simulink library "vmc"  (R2021b)
settings: Solver=VariableStepAuto  StartTime=0.0  StopTime=10.0  RelTol=1e-3
undefined symbols (not defined in the file or in its folder): AVMC_ACCDeltaTqIGain_X_kph, AVMC_ACCDeltaTqIGain_Y_mps2, AVMC_ACCDeltaTqIGainP2_X_kph, AVMC_ACCDeltaTqIGainP2_Y_mps2, AVMC_ACCDeltaTqPGain_X_kph, AVMC_ACCDeltaTqPGain_Y_kph, AVMC_ACCDeltaTqPGainP2_X_kph, AVMC_ACCDeltaTqPGainP2_Y_kph, AVMC_ACCLongSteadyCtrl_X_kph, AVMC_CCAccelCMD_X_kph, AVMC_CCAccelCMD_Y_kph, AVMC_CCDeltaTqIGain_X_kph, AVMC_CCDeltaTqIGain_Y_mps2, AVMC_CCDeltaTqPGain_X_kph, AVMC_CCDeltaTqPGain_Y_kph, AVMC_CCLongSteadyCtrl_X_kph, AVMC_DISCDeltaTqIGainP2_X_kph, AVMC_DISCDeltaTqIGainP2_Y_mps2, AVMC_ESCRegenOut_X_kph, AVMC_ESCRegenOut_Y_Deg, AVMC_ESCRegenOutEnSpd_X_Deg, AVMC_LatESCRegenOut_X_kph, AVMC_LatESCRegenOut_Y_Deg, AVMC_LongAccDeadZone_X_kph, AVMC_LongAccDeadZoneP2_X_kph, AVMC_LongAccFiltTs_X_Gps, AVMC_LongAccFiltTsP2_X_Gps, AVMC_MCPresBaseTq_X_bar, AVMC_MSAAccelCMD_X_kph, AVMC_MSAAccelCMD_Y_kph, AVMC_MSADeltaTqIGain_X_kph, AVMC_MSADeltaTqIGain_Y_mps2, AVMC_MSADeltaTqPGain_X_kph, AVMC_MSADeltaTqPGain_Y_kph, AVMC_MSALongSteadyCtrl_X_kph, AVMC_MSAPedalOvrd_X_kph, AVMC_MSASpdBand_X_kph, AVMC_OPDDisSlideRate_X_Deg, AVMC_RDCDetectTime_X_kph, AVMC_RDCDetectTime_Y_pct, AVMC_RDCEnSlideRate_X_Deg, AVMC_StESCYaw_X_kph, AVMC_StESCYaw_Y_Deg, AVMC_StESCYawCom_X_kph, AVMC_StESCYawCom_Y_Gps, AVMC_TMSpdBaseTq_X_rpm, C_TASK_10MS_S, C_TASK_5MS_S, DEG2RAD, Discrete, ENUM_ADASACCSTA_ACTIVE, ENUM_ADASACCSTA_OVERRIDE, ENUM_ADASACCSTA_STANDBY, ENUM_ADASMSASTA_ACTIVE, ENUM_ADASMSASTA_ERROR, ENUM_ADASMSASTA_OFF, ENUM_ADASMSASTA_OVERSPEED, ENUM_ADASMSASTA_STANDBY, ENUM_ADASMSASTA_UNDERSPEED, ENUM_ADASMSASTA_UNLIMIT ... (+254)
libraries: hcu_lib x57, simulink x49, ctrlSharedLib x6, simulink_extras x1
(part 7 of 9)

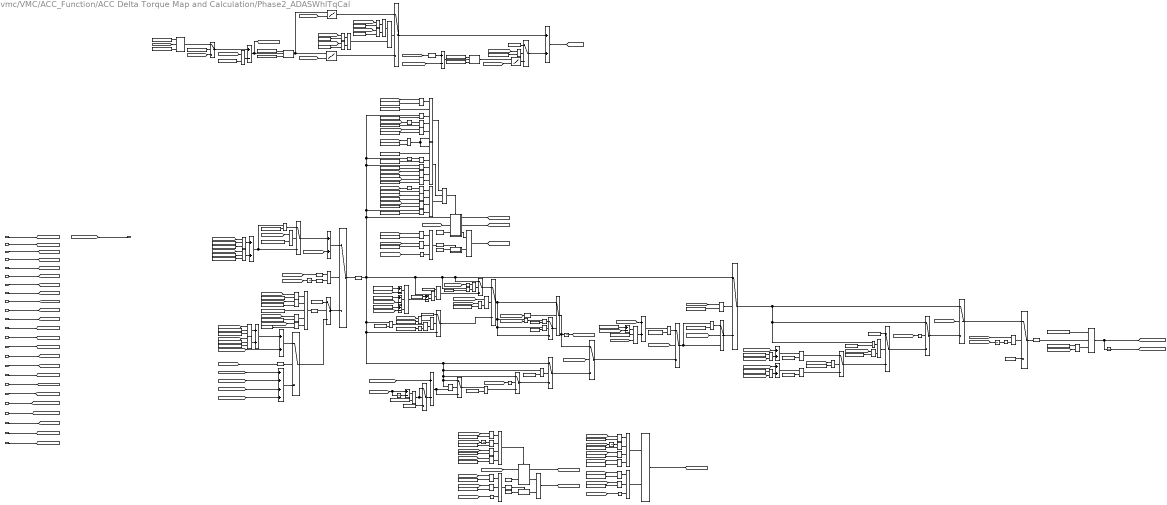
== system vmc/VMC/ACC_Function/ACC Delta Torque Map and Calculation/Phase2_ADASWhlTqCal ==
  note: Deceleration REGEN Torque Control
  note: Deceleration REGEN Torque Control Judgement
  note: Deceleration Torque Control
  note: Deceleration Positive Torque Control
  VVMC_TotalAvailBrkRgnTq_Nm : Inport
  VVMC_AccelTurnHold_flg : Inport  Port=2
  VVMC_ADASActive_flg : Inport  Port=3
  VVMC_ACCPedalOvrd_flg : Inport  Port=4
  task_time_s : Inport  Port=5
  VINP_ESCADASSta_enum : Inport  Port=6
  VVMC_MCPreBaseTqEn_flg : Inport  Port=7
  VINP_ACCVehHoldReq_flg : Inport  Port=8
  VINP_VehSpeed_kph : Inport  Port=9
  VINP_MCPressure_bar : Inport  Port=10
  VVMC_ADASNegReq_flg : Inport  Port=11
  VVMC_TimeGapJudge_flag : Inport  Port=12
  VTQR_FrTMTqReq_Nm : Inport  Port=13
  VTQR_RrTMTqReq_Nm : Inport  Port=14
  VVMC_LongAcc_Gps : Inport  Port=15
  VVMC_FeatSetSpdForCalcu_kph : Inport  Port=16
  VVMC_MeterIndSpeedForCalcu_kph : Inport  Port=17
  VINP_ADASACCSta_enum : Inport  Port=18
  VVMC_AfterCtrlACCReqAccel_mps2 : Inport  Port=19
  VVMC_TMSpdBaseTq_Nm : Inport  Port=20
  VVMC_MCPresBaseTq_Nm : Inport  Port=21
  VVMC_EstSlope_Deg : Inport  Port=22
  VVMC_ACCReqSpdMemory_kph : Inport  Port=23
  VVMC_ACCSpdCtrl_flg : Inport  Port=24
  AND{10,13,17,20,29,31} (6 alike) : Logic  AllPortsSameDT=off  OutDataTypeStr=boolean
  AND14 : Logic  Operator=OR  AllPortsSameDT=off  OutDataTypeStr=boolean
  AND19 : Logic  Operator=OR  AllPortsSameDT=off  OutDataTypeStr=boolean
  AND32 : Logic  Inputs=5  AllPortsSameDT=off  OutDataTypeStr=boolean
  Add{1,3,13,15,18..21} (8 alike) : Sum
  Add{4..5,7..12,14} (9 alike) : Sum  Inputs=+-
  Add6 : Sum  Inputs=++++
  Cast To Single2 : DataTypeConversion  OutDataTypeStr=single
  Cast To Single3 : DataTypeConversion  OutDataTypeStr=single
  Constant1 : Constant  Value=ENUM_ADASACCSTA_ACTIVE
  Constant10 : Constant  Value=KVMC_ADASWhlTqLowerLim_Nm
  Constant100 : Constant  Value=KVMC_ZeroRgnTqSpdCtrlTime_s
  Constant{30,42..43,46,48,53..56,58,63..64,66..67,69..70,72..75,81..82,87,89..90,92..93,96,98..99,101,112,114,116..117,124..125,131..132,151,156,163,168,170,174} (45 alike) : Constant  Value=ZERO_FLOAT
  Constant11 : Constant  Value=KVMC_ReqAccelLimitSW_flg
  Constant115 : Constant  Value=KVMC_ACCLowSpdPosTq_flg
  Constant12 : Constant  Value=KVMC_AccDevLowLim_mps2
  Constant13 : Constant  Value=KVMC_AccDevUpLim_mps2
  Constant14 : Constant  Value=KVMC_ACCSpdDevUpLim_kph
  Constant15 : Constant  Value=KVMC_ACCSpdDevLowLim_kph
  Constant157 : Constant  Value=KVMC_AccelTurnHoldZeroTq_flg
  Constant16 : Constant  Value=KVMC_ReqAccelUpperLimit_mps2
  Constant162 : Constant  Value=KVMC_HoldTqRamp2ZeroSlope_Nmps
  Constant166 : Constant  Value=ENUM_ESCADASSTA_VEHASTANDSTILL
  Constant167 : Constant  Value=KVMC_StandstillTqRamp2ZeroSlope_Nmps
  Constant17 : Constant  Value=KVMC_ReqAccelLowerLimit_mps2
  Constant171 : Constant  Value=KVMC_BigDeltaDecGapBand_mps2
  Constant172 : Constant  Value=KVMC_BigDeltaDecJudgeEnBand_mps2
  Constant173 : Constant  Value=KVMC_BigDeltaDecEnGradeBand_deg
  Constant2 : Constant  Value=KTQR_FrTMGearEff_c
  Constant23 : Constant  Value=TRUE
  Constant27 : Constant  Value=KVMC_TimeGapTq2Zero_flg
  Constant3 : Constant  Value=KTQD_FrTMTotalGearRatio_gain
  Constant{38..39,57,62,77,80,88,97} (8 alike) : Constant  Value=KVMC_CutOffNegTqSpd_kph
  Constant4 : Constant  Value=KTQD_RrTMTotalGearRatio_gain
  Constant40 : Constant  Value=KTQR_FrTMGearEff_c
  Constant41 : Constant  Value=FALSE
  Constant{44,50..51,78..79,91} (6 alike) : Constant  Value=KVMC_ZeroRgnTqSpd_kph
  Constant45 : Constant  Value=KTQD_FrTMTotalGearRatio_gain
  Constant5 : Constant  Value=KTQR_RrTMGearEff_c
  Constant59 : Constant  Value=KVMC_TqMCPRelFactor_Nm
  Constant68 : Constant  Value=KVMC_GradeTqCtrl_flg
  Constant71 : Constant  Value=KVMC_BigDeltaDecGapZeroTq_flg
  Constant76 : Constant  Value=KVMC_DownGradeTqCtrl_flg
  Constant8 : Constant  Value=KVMC_ADASWhlTqUpperLim_Nm
  Constant84 : Constant  Value=KTQD_RrTMTotalGearRatio_gain
  Constant85 : Constant  Value=KTQR_RrTMGearEff_c
  Constant9 : Constant  Value=KVMC_GravityValue_mps2
  Constant94 : Constant  Value=TRUE
  Constant95 : Constant  Value=FALSE
  Data Type Conversion1 : DataTypeConversion  OutDataTypeStr=single
  Detect Decrease2 : simulink/Logic and Bit Operations/Detect Decrease  vinit=0.0  OutDataTypeStr=boolean
  Detect Decrease3 : simulink/Logic and Bit Operations/Detect Decrease  vinit=0.0  OutDataTypeStr=boolean
  Detect Increase{3..5,7..8} (5 alike) : simulink/Logic and Bit Operations/Detect Increase  vinit=0.0  OutDataTypeStr=boolean
  Divide : Product  Inputs=*/*
  Divide{1,4..5,8} (4 alike) : Product  Inputs=***
  Divide2 : Product  Inputs=**
  Divide3 : Product  Inputs=*/*
  Divide6 : Product  Inputs=**
  Divide7 : Product  Inputs=**
  Equal10 : RelationalOperator  Operator===  OutDataTypeStr=boolean  RndMeth=Simplest
  Equal11 : RelationalOperator  Operator=<  OutDataTypeStr=boolean  RndMeth=Simplest
  Equal12 : RelationalOperator  Operator=>  OutDataTypeStr=boolean  RndMeth=Simplest
  Equal6 : RelationalOperator  Operator=<  OutDataTypeStr=boolean  RndMeth=Simplest
  Equal7 : RelationalOperator  Operator=>  OutDataTypeStr=boolean  RndMeth=Simplest
  Equal8 : RelationalOperator  Operator=<  OutDataTypeStr=boolean  RndMeth=Simplest
  Equal9 : RelationalOperator  Operator=>  OutDataTypeStr=boolean  RndMeth=Simplest
  InitialCondition: 1 : UnitDelay  SampleTime=-1  HasFrameUpgradeWarning=on
  Logical Operator1 : Logic  Inputs=4  AllPortsSameDT=off  OutDataTypeStr=boolean
  Logical Operator10 : Logic  Operator=OR  Inputs=3  AllPortsSameDT=off  OutDataTypeStr=boolean
  Logical Operator2 : Logic  Operator=OR  AllPortsSameDT=off  OutDataTypeStr=boolean
  Logical Operator3 : Logic  Inputs=6  AllPortsSameDT=off  OutDataTypeStr=boolean
  Logical Operator4 : Logic  Operator=OR  Inputs=3  AllPortsSameDT=off  OutDataTypeStr=boolean
  Logical Operator5 : Logic  Inputs=6  AllPortsSameDT=off  OutDataTypeStr=boolean
  Logical Operator6 : Logic  AllPortsSameDT=off  OutDataTypeStr=boolean
  Logical Operator7 : Logic  Inputs=4  AllPortsSameDT=off  OutDataTypeStr=boolean
  Logical Operator8 : Logic  Operator=OR  Inputs=3  AllPortsSameDT=off  OutDataTypeStr=boolean
  Logical Operator9 : Logic  Inputs=4  AllPortsSameDT=off  OutDataTypeStr=boolean
  MVMC_ACCDeltaTqIGain_Z_Nm : Lookup_n-D  BreakpointsForDimension1=AVMC_ACCDeltaTqIGainP2_Y_mps2  BreakpointsForDimension2=AVMC_ACCDeltaTqIGainP2_X_kph  Table=MVMC_ACCDeltaTqIGainP2_Z_Nm  InternalRulePriority=Speed  RndMeth=Simplest  InputSameDT=on
      settings: InputPortMap=u0,u1
  MVMC_ACCDeltaTqPGain_Z_Nm1 : Lookup_n-D  BreakpointsForDimension1=AVMC_ACCDeltaTqPGainP2_Y_kph  BreakpointsForDimension2=AVMC_ACCDeltaTqPGainP2_X_kph  Table=MVMC_ACCDeltaTqPGainP2_Z_Nm  InternalRulePriority=Speed  RndMeth=Simplest  InputSameDT=on
      settings: InputPortMap=u0,u1
  MVMC_DISCDeltaTqIGain_Z_Nm : Lookup_n-D  BreakpointsForDimension1=AVMC_DISCDeltaTqIGainP2_Y_mps2  BreakpointsForDimension2=AVMC_DISCDeltaTqIGainP2_X_kph  Table=MVMC_DISCDeltaTqIGainP2_Z_Nm  InternalRulePriority=Speed  RndMeth=Simplest  InputSameDT=on
      settings: InputPortMap=u0,u1
  Max{,1,4..5,7..8} (6 alike) : MinMax  Function=max  Inputs=2
  Max2 : MinMax  Inputs=2
  Max3 : MinMax  Inputs=2
  Merge : Merge
  Merge2 : Merge
  Min : MinMax  Inputs=2
  Min1 : MinMax  Inputs=2
  Min2 : MinMax  Function=max  Inputs=2
  NOT{1,4..6,9,12..13,15} (8 alike) : Logic  Operator=NOT  AllPortsSameDT=off  OutDataTypeStr=boolean
  OR18 : Logic  Operator=OR  AllPortsSameDT=off  OutDataTypeStr=boolean
  OR2 : Logic  Operator=OR  Inputs=3  AllPortsSameDT=off  OutDataTypeStr=boolean
  OR5 : Logic  AllPortsSameDT=off  OutDataTypeStr=boolean
  Product1 : Product
  Relational Operator1 : RelationalOperator  Operator=~=  OutDataTypeStr=boolean  RndMeth=Simplest
  Relational Operator{2,10,12,24..25,29,36..37,39,42..43} (11 alike) : RelationalOperator  OutDataTypeStr=boolean  RndMeth=Simplest
  Relational Operator{9,11,14..15,21..23,26,28,30..31,35,41,45,49..50} (16 alike) : RelationalOperator  Operator=<  OutDataTypeStr=boolean  RndMeth=Simplest
  Relational Operator{20,27,34,40,71,74} (6 alike) : RelationalOperator  Operator=<=  OutDataTypeStr=boolean  RndMeth=Simplest
  Relational Operator{32..33,38,44,47} (5 alike) : RelationalOperator  Operator=>  OutDataTypeStr=boolean  RndMeth=Simplest
  SR_Latch : hcu_lib/Basic_Blocks/SR_Latch
  Saturation Dynamic{1..3,5} (4 alike) : simulink/Discontinuities/Saturation Dynamic  OutMin=[]  OutMax=[]  OutDataTypeStr=Inherit: Same as second input  OutDataType=fixdt(1, 16)  OutScaling=2^-10  DoSatur=off
  Switch{,1,4,7..8,10,12..19,21..24,27,29,33..34,39,41,43} (25 alike) : Switch  Criteria=u2 > Threshold
  Triggered Subsystem1 : Subsystem  TreatAsAtomicUnit=on
  Triggered Subsystem2 : Subsystem  TreatAsAtomicUnit=on
  Triggered Subsystem4 : Subsystem  TreatAsAtomicUnit=on
  Triggered Subsystem5 : Subsystem  TreatAsAtomicUnit=on
  Unit Delay{1..5,7..9,11} (9 alike) : UnitDelay  SampleTime=-1  HasFrameUpgradeWarning=on
  VVMC_ADASWhlTqCal_Nm : Outport
  wires:
  Constant66/1 -> Relational Operator23/2
  Relational Operator42/1 -> Logical Operator9/2
  Detect Increase3/1 -> Triggered Subsystem2/Trigger
  Detect Decrease3/1 -> Logical Operator2/2
  Unit Delay2/1 -> Detect Decrease3/1
  NOT13/1 -> AND10/1
  Max2/1 -> Switch24/1
  Relational Operator30/1 -> Logical Operator5/3
  Relational Operator44/1 -> Logical Operator10/1
  [VTQR_RrTMTqReq_Nm] -> Divide5/1
  Constant162/1 -> Divide6/1
  NOT6/1 -> OR5/2
  Switch19/1 -> Switch18/3
  Relational Operator47/1 -> AND10/2
  Constant112/1 -> Relational Operator47/2
  Max4/1 -> Min1/2
  Constant99/1 -> Add14/1
  Constant68/1 -> Logical Operator3/2
  [VVMC_ACCLowSpdCtrlEnSpd_kph] -> Relational Operator33/1
  NOT15/1 -> Logical Operator10/3
  Constant39/1 -> Relational Operator12/2
  Constant77/1 -> Relational Operator31/2
  Merge2/1 -> [VVMC_ZeroRgnTqSpdCtrl_flg]  "VVMC_ZeroRgnTqSpdCtrl_flg"
  Relational Operator38/1 -> Logical Operator8/1
  Switch17/1 -> Relational Operator71/1, Switch13/1, Switch4/1
  Constant115/1 -> NOT12/1
  Constant46/1 -> Min/2
  [VVMC_ActACCRequiredAccel_mps2] -> Unit Delay7/1
  Cast To Single2/1 -> Relational Operator9/1, Switch10/1, Switch16/1, Relational Operator26/1, Switch19/1, Switch21/3, Relational Operator49/1, Relational Operator30/1, Unit Delay4/1, Relational Operator23/1, Relational Operator15/1, Triggered Subsystem1/1(In1), Max4/1, Relational Operator47/1, Switch27/1, Switch17/1  "VVMC_OriADASWhlTqP2_Nm"
  Relational Operator39/1 -> Logical Operator7/1
  Unit Delay8/1 -> [VVMC_LastACCLowSpdTq_Nm]
  Divide6/1 -> Add20/2
  [VVMC_ZeroRgnTqSpdCtrlTq_Nm] -> Add14/2
  Constant93/1 -> Relational Operator42/2
  Relational Operator22/1 -> Logical Operator3/6
  Constant44/1 -> Relational Operator20/2
  Relational Operator27/1 -> AND32/1
  Add9/1 -> Divide/2
  Constant90/1 -> Relational Operator39/2
  Equal10/1 -> Switch41/2
  Add21/1 -> Max8/1
  [VVMC_ADASActive_flg] -> NOT4/1
  Add14/1 -> Divide3/1
  Switch41/1 -> Switch39/3
  Relational Operator43/1 -> Logical Operator10/2
  Detect Increase5/1 -> Switch22/2
  [VVMC_LastADASWhlTqCal_Nm] -> Relational Operator39/1
  InitialCondition: 1/1 -> [VVMC_LastADASWhlTqCal_Nm]  "VVMC_LastADASWhlTqCalP2_Nm"
  Relational Operator12/1 -> Logical Operator1/1
  OR2/1 -> Triggered Subsystem1/Trigger
  Divide3/1 -> Add15/2
  Constant151/1 -> Relational Operator71/2
  Triggered Subsystem1/3(Out3) -> Merge/1
  [VINP_VehSpeed_kph] -> Relational Operator38/1
  Add8/1 -> Divide/1
  AND29/1 -> OR18/2
  Constant95/1 -> Triggered Subsystem5/1(In1)
  Constant97/1 -> Relational Operator44/2
  Max3/1 -> Switch29/1
  Detect Increase8/1 -> Switch43/2
  [VVMC_ActACCRequiredAccel_mps2] -> Relational Operator43/1
  Triggered Subsystem2/1(Out1) -> Merge/2
  Constant89/1 -> Max1/2
  [VVMC_ADASActive_flg] -> NOT15/1
  Switch39/1 -> Switch13/3
  Triggered Subsystem5/1(Out1) -> Merge2/2
  Constant53/1 -> Add10/1
  Switch23/1 -> Switch17/3
  Relational Operator28/1 -> Logical Operator5/5
  Constant57/1 -> Relational Operator2/2
  Constant98/1 -> Relational Operator45/2
  [VVMC_ActACCRequiredAccel_mps2] -> Relational Operator14/1
  Add18/1 -> Switch8/1
  Constant48/1 -> Relational Operator15/2
  Switch43/1 -> Switch8/3
  [task_time_s] -> Divide7/2
  AND31/1 -> Switch33/2
  Switch33/1 -> Add18/1
  [VVMC_ADASActive_flg] -> Detect Increase4/1
  [VTQR_FrTMTqReq_Nm] -> Divide1/1
  Switch4/1 -> Switch7/1
  Relational Operator32/1 -> Logical Operator5/6, Logical Operator3/1
  [VINP_VehSpeed_kph] -> Relational Operator44/1
  AND10/1 -> Switch27/2
  [VVMC_ActACCRequiredAccel_mps2] -> Relational Operator28/1
  [VVMC_ADASNegReq_flg] -> NOT13/1
  [VINP_VehSpeed_kph] -> Relational Operator2/1
  [VVMC_ActACCRequiredAccel_mps2] -> Relational Operator22/1
  Relational Operator29/1 -> Logical Operator5/4
  Add20/1 -> Max7/1
  NOT9/1 -> Logical Operator8/3
  [VVMC_ACCPedalOvrd_flg] -> Unit Delay2/1
  Relational Operator45/1 -> Logical Operator9/1
  [VINP_VehSpeed_kph] -> Unit Delay1/1
  [VVMC_AccelTurnHold_flg] -> AND29/1
  AND14/1 -> AND13/2
  Max8/1 -> Switch41/1
  [VINP_ESCADASSta_enum] -> Equal10/1
  Constant96/1 -> Relational Operator43/2
  [VINP_VehSpeed_kph] -> Relational Operator32/1
  Constant114/1 -> Relational Operator49/2
  [VVMC_EstSlope_Deg] -> Equal11/1
  Max/1 -> Max3/1
  Constant116/1 -> Relational Operator50/2
  Constant73/1 -> Relational Operator29/2
  Relational Operator15/1 -> Logical Operator1/4
  Switch21/1 -> Switch12/3
  Constant172/1 -> Relational Operator74/2
  Constant84/1 -> Divide5/2
  Constant92/1 -> Relational Operator41/2
  Unit Delay1/1 -> Relational Operator12/1
  Divide5/1 -> Add13/2
  Logical Operator10/1 -> Detect Increase7/1
  [VVMC_ACCLowSpdTqCtrl_flg] -> Detect Increase5/1
  Triggered Subsystem1/1(Out1) -> [VVMC_ACCLowSpdTqLimit_Nm]  "VVMC_ACCLowSpdTqLimit_Nm"
  Saturation Dynamic2/1 -> [VVMC_ADASWhlTqCal_Nm], InitialCondition: 1/1  "VVMC_ADASWhlTqCalP2_Nm"
  OR5/1 -> Switch7/2
  Relational Operator33/1 -> Logical Operator6/2
  Divide/1 -> Add4/2
  Relational Operator50/1 -> Switch29/2
  Min1/1 -> Switch27/3
  [VVMC_ActACCRequiredAccel_mps2] -> Relational Operator37/1
  Add6/1 -> Switch14/3
  Logical Operator2/1 -> Switch8/2
  Switch29/1 -> Switch22/3
  OR18/1 -> Switch39/2
  Logical Operator6/1 -> Switch12/2
  Constant170/1 -> Switch43/1
  Switch8/1 -> Cast To Single2/1
  Constant80/1 -> Relational Operator34/2
  Constant42/1 -> Relational Operator24/2
  Unit Delay9/1 -> Relational Operator36/1
  [VINP_VehSpeed_kph] -> Relational Operator20/1
  Relational Operator74/1 -> AND32/2
  Relational Operator41/1 -> Logical Operator9/3
  Switch12/1 -> Switch29/3, Relational Operator50/1, Max/1, Switch22/1
  Relational Operator36/1 -> Logical Operator7/2
  [VINP_VehSpeed_kph] -> Relational Operator11/1
  [VVMC_TimeGapJudge_flag] -> AND31/1
  NOT4/1 -> Logical Operator4/3
  [task_time_s] -> Divide3/3
  Relational Operator71/1 -> OR18/1
  Constant75/1 -> Relational Operator30/2
  [VINP_VehSpeed_kph] -> Relational Operator31/1
  [VINP_VehSpeed_kph] -> Relational Operator34/1
  Relational Operator49/1 -> AND14/1
  Constant76/1 -> Logical Operator5/2
  Constant166/1 -> Equal10/2
  Detect Increase4/1 -> Logical Operator2/1
  Constant74/1 -> Switch7/3
  Constant64/1 -> Relational Operator22/2
  Constant40/1 -> Divide1/3
  Divide7/1 -> Add21/2
  [VINP_VehSpeed_kph] -> Relational Operator21/1
  Logical Operator3/1 -> OR2/2
  Constant163/1 -> Max7/2
  Constant54/1 -> Add4/1
  [task_time_s] -> Divide6/2
  Constant82/1 -> Relational Operator36/2
  [VINP_ACCVehHoldReq_flg] -> NOT5/1
  [VVMC_LastADASWhlTqCal_Nm] -> Add15/1
  Constant117/1 -> Max3/2
  [VVMC_ZeroRgnTqSpdCtrl_flg] -> Switch24/2
  Constant56/1 -> Switch21/1
  Constant23/1 -> Triggered Subsystem1/3(In3)
  [VINP_VehSpeed_kph] -> Relational Operator40/1
  Switch7/1 -> Cast To Single3/1
  Constant71/1 -> AND32/3
  Constant157/1 -> AND29/2
  [VVMC_ACCLowSpdCtrlEnSpd_kph] -> Add9/2
  NOT12/1 -> AND14/2
  Constant167/1 -> Divide7/1
  Constant55/1 -> Min1/1
  [VVMC_ActACCRequiredAccel_mps2] -> Relational Operator24/1
  Relational Operator31/1 -> Logical Operator5/1
  Logical Operator5/1 -> OR2/1
  Constant78/1 -> Relational Operator32/2
  Constant100/1 -> Divide3/2
  [VVMC_ACCDeltaTq_Nm] -> Add19/2
  [VVMC_MCPresBaseTq_Nm] -> Add6/4
  Constant101/1 -> Max2/2
  Constant174/1 -> Equal12/2
  Constant85/1 -> Divide5/3
  AND13/1 -> Switch21/2
  [VVMC_ACCDeltaTq_Nm] -> Add18/2
  [VVMC_TMSpdBaseTq_Nm] -> Add6/3
  Relational Operator37/1 -> Logical Operator8/2
  Relational Operator2/1 -> Logical Operator4/1
  Constant72/1 -> Relational Operator28/2
  Constant87/1 -> Relational Operator37/2
  AND32/1 -> Detect Increase8/1
  [VVMC_LastADASWhlTqCal_Nm] -> Add6/1
  Triggered Subsystem1/2(Out2) -> [VVMC_ACCLowSpdCtrlEnSpd_kph]  "VVMC_ACCLowSpdCtrlEnSpd_kph"
  Constant168/1 -> Max8/2
  Switch24/1 -> Switch23/3, Max1/1
  [VVMC_ACCPedalOvrd_flg] -> Unit Delay5/1
  Merge/1 -> [VVMC_ACCLowSpdTqCtrl_flg]  "VVMC_ACCLowSpdTqCtrl_flg"
  Relational Operator21/1 -> Logical Operator3/5
  Relational Operator24/1 -> Switch17/2
  Constant27/1 -> AND31/2
  Constant171/1 -> Relational Operator27/2
  Max7/1 -> Switch41/3
  [VVMC_ACCLowSpdTqCtrl_flg] -> Logical Operator6/1
  Constant156/1 -> Switch39/1
  Relational Operator35/1 -> Logical Operator7/3
  Switch27/1 -> Switch12/1
  [VVMC_ACCDeltaAccel_mps2] -> Relational Operator27/1
  Relational Operator11/1 -> Logical Operator1/2
  Relational Operator20/1 -> AND13/1
  [VVMC_LastADASWhlTqCal_Nm] -> Equal12/1
  [VVMC_LastADASWhlTqCal_Nm] -> Add21/1
  [VVMC_ADASActive_flg] -> NOT9/1
  [VVMC_LastACCLowSpdTq_Nm] -> Max/2
  [VVMC_RgnProhibited_flg] -> Switch23/2
  [VVMC_ActACCRequiredAccel_mps2] -> Unit Delay9/1
  [VVMC_LastADASWhlTqCal_Nm] -> Triggered Subsystem4/1(In1)
  Unit Delay7/1 -> Relational Operator29/1
  Switch22/1 -> Switch18/1, Unit Delay8/1  "VVMC_ACCLowSpdTq_Nm"
  Equal12/1 -> AND32/5
  Relational Operator25/1 -> Logical Operator3/3
  Constant81/1 -> Relational Operator35/2
  [VVMC_ActACCRequiredAccel_mps2] -> Relational Operator74/1
  Detect Decrease2/1 -> Switch14/2
  Triggered Subsystem4/2(Out2) -> Merge2/1
  [VVMC_ACCLowSpdTqCtrl_flg] -> Switch18/2
  Equal11/1 -> AND32/4
  [VVMC_ActACCRequiredAccel_mps2] -> Relational Operator35/1
  Constant43/1 -> Relational Operator14/2
  Switch13/1 -> Switch4/3
  Constant88/1 -> Relational Operator38/2
  [VVMC_ACCDeltaTq_Nm] -> Add6/2
  Relational Operator14/1 -> Logical Operator1/3
  [VVMC_MCPreBaseTqEn_flg] -> Switch4/2
  [VVMC_LastADASWhlTqCal_Nm] -> Add20/1
  Constant51/1 -> Add9/1
  [VVMC_ADASActive_flg] -> OR5/1
  Constant62/1 -> Relational Operator21/2
  [VVMC_ACCLowSpdTqLimit_Nm] -> Add10/2
  Add13/1 -> Min/1, Switch33/3
  SR_Latch/1 -> [VVMC_RgnProhibited_flg]  "VVMC_RgnProhibited_flg"
  Relational Operator40/1 -> Logical Operator9/4
  Triggered Subsystem4/1(Out1) -> [VVMC_ZeroRgnTqSpdCtrlTq_Nm]  "VVMC_ZeroRgnTqSpdCtrlTq_Nm"
  Relational Operator23/1 -> Logical Operator3/4
  Unit Delay4/1 -> Relational Operator25/1
  [VVMC_ActACCRequiredAccel_mps2] -> Relational Operator10/1
  [VINP_VehSpeed_kph] -> Triggered Subsystem1/2(In2)
  [VVMC_ActACCRequiredAccel_mps2] -> Unit Delay11/1
  Constant79/1 -> Relational Operator33/2
  Logical Operator4/1 -> Detect Increase3/1
  Logical Operator9/1 -> Triggered Subsystem4/Trigger
  Constant173/1 -> Equal11/2
  Constant41/1 -> Triggered Subsystem2/1(In1)
  Add4/1 -> Max4/2
  Divide1/1 -> Add13/1
  Constant91/1 -> Relational Operator40/2
  Add15/1 -> Max2/1
  Unit Delay11/1 -> Relational Operator42/1
  [VVMC_LastADASWhlTqCal_Nm] -> Relational Operator45/1
  Max1/1 -> Switch23/1
  Constant45/1 -> Divide1/2
  Switch14/1 -> Switch43/3
  Relational Operator34/1 -> Logical Operator7/4
  Add10/1 -> Divide/3
  Switch18/1 -> Switch24/3
  [VINP_VehSpeed_kph] -> Add8/2
  Constant94/1 -> Triggered Subsystem4/2(In2)
  NOT5/1 -> Switch13/2
  Constant67/1 -> Relational Operator25/2
  Add19/1 -> Switch14/1
  Constant50/1 -> Add8/1
  Detect Increase7/1 -> Triggered Subsystem5/Trigger
  Constant30/1 -> Relational Operator10/2
  Unit Delay5/1 -> NOT6/1
  Logical Operator1/1 -> OR2/3
  Relational Operator10/1 -> Logical Operator4/2
  Constant38/1 -> Relational Operator11/2
  [VVMC_ActACCRequiredAccel_mps2] -> Relational Operator41/1
  [VVMC_ADASNegReq_flg] -> Detect Decrease2/1
  VVMC_AccelTurnHold_flg/1 -> [VVMC_AccelTurnHold_flg]
  VVMC_TotalAvailBrkRgnTq_Nm/1 -> [VVMC_TotalAvailBrkRgnTq_Nm]
  [VVMC_ADASWhlTqCal_Nm] -> VVMC_ADASWhlTqCal_Nm/1
  VVMC_ADASActive_flg/1 -> [VVMC_ADASActive_flg]
  VVMC_ACCPedalOvrd_flg/1 -> [VVMC_ACCPedalOvrd_flg]
  task_time_s/1 -> [task_time_s]
  VINP_ESCADASSta_enum/1 -> [VINP_ESCADASSta_enum]
  VVMC_MCPreBaseTqEn_flg/1 -> [VVMC_MCPreBaseTqEn_flg]
  VINP_ACCVehHoldReq_flg/1 -> [VINP_ACCVehHoldReq_flg]
  VINP_VehSpeed_kph/1 -> [VINP_VehSpeed_kph]
  VINP_MCPressure_bar/1 -> [VINP_MCPressure_bar]
  VVMC_ADASNegReq_flg/1 -> [VVMC_ADASNegReq_flg]
  VVMC_TimeGapJudge_flag/1 -> [VVMC_TimeGapJudge_flag]
  VTQR_FrTMTqReq_Nm/1 -> [VTQR_FrTMTqReq_Nm]
  VTQR_RrTMTqReq_Nm/1 -> [VTQR_RrTMTqReq_Nm]
  Saturation Dynamic1/1 -> MVMC_DISCDeltaTqIGain_Z_Nm/1, MVMC_ACCDeltaTqIGain_Z_Nm/1  "VVMC_ActAccDevP2_mps2"
  Saturation Dynamic5/1 -> MVMC_ACCDeltaTqPGain_Z_Nm1/1  "VVMC_ACCActSpdDevP2_kph"
  MVMC_ACCDeltaTqPGain_Z_Nm1/1 -> Switch1/3
  AND20/1 -> AND19/2
  Constant9/1 -> Product1/2
  Constant12/1 -> Saturation Dynamic1/3
  Switch1/1 -> Add3/2  "VVMC_ACCDeltaTqPGainP2_Nm"
  Constant58/1 -> Switch1/1
  Relational Operator1/1 -> Switch1/2
  Add5/1 -> Saturation Dynamic5/2
  Data Type Conversion1/1 -> Add5/1
  [VVMC_ActACCRequiredAccel_mps2] -> Equal7/1
  [VVMC_LongAcc_Gps] -> Equal6/1
  [VVMC_MeterIndSpeedForCalcu_kph] -> Add5/2
  Constant15/1 -> Saturation Dynamic5/3
  [VVMC_FeatSetSpdForCalcu_kph] -> Data Type Conversion1/1
  AND19/1 -> Switch34/2
  [VINP_VehSpeed_kph] -> MVMC_ACCDeltaTqPGain_Z_Nm1/2
  Product1/1 -> Add7/2
  Constant131/1 -> Equal8/2
  Constant124/1 -> Equal6/2
  [VINP_VehSpeed_kph] -> MVMC_DISCDeltaTqIGain_Z_Nm/2
  Add7/1 -> [VVMC_ACCDeltaAccel_mps2], Saturation Dynamic1/2
  [VVMC_ACCDeltaAccel_mps2] -> Equal9/1
  Constant132/1 -> Equal9/2
  [VVMC_LongAcc_Gps] -> Product1/1
  Equal7/1 -> AND17/2
  Constant125/1 -> Equal7/2
  MVMC_DISCDeltaTqIGain_Z_Nm/1 -> Switch34/1
  MVMC_ACCDeltaTqIGain_Z_Nm/1 -> Switch34/3
  Constant14/1 -> Saturation Dynamic5/1
  [VVMC_ActACCRequiredAccel_mps2] -> Switch/3
  Switch34/1 -> Add3/1  "VVMC_ACCDeltaTqIGainP2_Nm"
  [VINP_VehSpeed_kph] -> MVMC_ACCDeltaTqIGain_Z_Nm/2
  Equal6/1 -> AND17/1
  Equal8/1 -> AND20/1
  Constant13/1 -> Saturation Dynamic1/1
  AND17/1 -> AND19/1
  Equal9/1 -> AND20/2
  Add3/1 -> [VVMC_ACCDeltaTq_Nm]  "VVMC_ACCDeltaTqP2_Nm"
  [VVMC_ActACCRequiredAccel_mps2] -> Equal8/1
  Constant1/1 -> Relational Operator1/2
  [VINP_ADASACCSta_enum] -> Relational Operator1/1
  VVMC_LongAcc_Gps/1 -> [VVMC_LongAcc_Gps]
  VVMC_FeatSetSpdForCalcu_kph/1 -> [VVMC_FeatSetSpdForCalcu_kph]
  VVMC_MeterIndSpeedForCalcu_kph/1 -> [VVMC_MeterIndSpeedForCalcu_kph]
  VINP_ADASACCSta_enum/1 -> [VINP_ADASACCSta_enum]
  VVMC_AfterCtrlACCReqAccel_mps2/1 -> [VVMC_ActACCRequiredAccel_mps2]
  VVMC_TMSpdBaseTq_Nm/1 -> [VVMC_TMSpdBaseTq_Nm]
  VVMC_MCPresBaseTq_Nm/1 -> [VVMC_MCPresBaseTq_Nm]
  Constant3/1 -> Divide4/2
  Divide4/1 -> Add1/1
  Constant5/1 -> Divide8/3
  Constant2/1 -> Divide4/3
  Divide8/1 -> Add1/2
  Constant4/1 -> Divide8/2
  [VTQR_FrTMTqReq_Nm] -> Divide4/1
  [VTQR_RrTMTqReq_Nm] -> Divide8/1
  Add1/1 -> Add19/1
  VVMC_EstSlope_Deg/1 -> [VVMC_EstSlope_Deg]
  VVMC_ACCReqSpdMemory_kph/1 -> [VVMC_ACCReqSpdMemory_kph]
  VVMC_ACCSpdCtrl_flg/1 -> [VVMC_ACCSpdCtrl_flg]
  [VVMC_TotalAvailBrkRgnTq_Nm] -> Max5/2
  Constant10/1 -> Max5/1
  Max5/1 -> Saturation Dynamic2/3
  Constant8/1 -> Saturation Dynamic2/1
  Cast To Single3/1 -> Saturation Dynamic2/2
  Constant11/1 -> Switch/2
  Switch/1 -> Add7/1
  Saturation Dynamic3/1 -> Switch/1
  [VVMC_ActACCRequiredAccel_mps2] -> Saturation Dynamic3/2
  Constant16/1 -> Saturation Dynamic3/1
  Constant17/1 -> Saturation Dynamic3/3
  Min/1 -> Switch33/1
  Relational Operator26/1 -> Switch19/2
  [VINP_MCPressure_bar] -> Add11/1, Unit Delay3/1
  Constant59/1 -> Divide2/2
  Constant69/1 -> Switch15/3
  [VVMC_ADASNegReq_flg] -> NOT1/1
  Switch16/1 -> Switch19/3
  Min2/1 -> Switch16/3
  Unit Delay3/1 -> Add11/2
  Constant63/1 -> Min2/2
  Switch15/1 -> Add12/2
  Switch10/1 -> Min2/1
  Constant70/1 -> Relational Operator26/2
  NOT1/1 -> Switch16/2
  Divide2/1 -> Switch15/1, Switch15/2
  Relational Operator9/1 -> Switch10/2
  Add12/1 -> Relational Operator9/2, Switch10/3  "VVMC_ACCTqRampOutByMCP_Nm"
  Add11/1 -> Divide2/1
  [VVMC_LastADASWhlTqCal_Nm] -> Add12/1
  Logical Operator7/1 -> SR_Latch/1
  Logical Operator8/1 -> SR_Latch/2

== system vmc/VMC/ACC_Function/ACC Torque Source Determination/Triggered Subsystem2 ==
  In1 : Inport
  Trigger : TriggerPort  VariantControl=(inherit)
  Out1 : Outport
  wires:
  In1/1 -> Out1/1

== system vmc/VMC/APS function/Signal Rounting/Signal Determination VINP_APSDecReqAtest_flg ==
  SignalInput1 : Inport
  SignalInput2 : Inport  Port=2
  VINP_SCPSystemMode_enum : Inport  Port=3
  VVMC_APSActive_flg : Inport  Port=4
  VVMC_ADASActive_flg : Inport  Port=5
  VVMC_CAASActive_flg : Inport  Port=6
  AND : Logic  Inputs=3  AllPortsSameDT=off  OutDataTypeStr=boolean
  Constant1 : Constant  Value=ENUM_SYSMODE_PRODUCT
  Constant3 : Constant  Value=KVMC_APSDevelopeSW_flg
  Equal : RelationalOperator  Operator===  OutDataTypeStr=boolean  RndMeth=Simplest
  OR : Logic  Operator=OR  Inputs=3  AllPortsSameDT=off  OutDataTypeStr=boolean
  Switch : Switch  Criteria=u2 > Threshold
  SignalOutp : Outport
  wires:
  VVMC_ADASActive_flg/1 -> OR/2
  AND/1 -> OR/1
  OR/1 -> Switch/2
  VVMC_APSActive_flg/1 -> AND/3
  Equal/1 -> AND/1
  VINP_SCPSystemMode_enum/1 -> Equal/1
  Switch/1 -> SignalOutp/1
  SignalInput1/1 -> Switch/1
  SignalInput2/1 -> Switch/3
  Constant3/1 -> AND/2
  Constant1/1 -> Equal/2
  VVMC_CAASActive_flg/1 -> OR/3

== system vmc/VMC/APS function/Signal Rounting/Signal Determination VINP_APSDecReqtest_mps2 ==
  SignalInput1 : Inport
  SignalInput2 : Inport  Port=2
  VINP_SCPSystemMode_enum : Inport  Port=3
  VVMC_APSActive_flg : Inport  Port=4
  VVMC_ADASActive_flg : Inport  Port=5
  VVMC_CAASActive_flg : Inport  Port=6
  AND : Logic  Inputs=3  AllPortsSameDT=off  OutDataTypeStr=boolean
  Constant1 : Constant  Value=ENUM_SYSMODE_PRODUCT
  Constant3 : Constant  Value=KVMC_APSDevelopeSW_flg
  Equal : RelationalOperator  Operator===  OutDataTypeStr=boolean  RndMeth=Simplest
  OR : Logic  Operator=OR  Inputs=3  AllPortsSameDT=off  OutDataTypeStr=boolean
  Switch : Switch  Criteria=u2 > Threshold
  SignalOutp : Outport
  wires:
  Constant1/1 -> Equal/2
  Constant3/1 -> AND/2
  SignalInput2/1 -> Switch/3
  SignalInput1/1 -> Switch/1
  Switch/1 -> SignalOutp/1
  VINP_SCPSystemMode_enum/1 -> Equal/1
  Equal/1 -> AND/1
  VVMC_APSActive_flg/1 -> AND/3
  OR/1 -> Switch/2
  AND/1 -> OR/1
  VVMC_ADASActive_flg/1 -> OR/2
  VVMC_CAASActive_flg/1 -> OR/3

== system vmc/VMC/APS function/Signal Rounting/Signal Determination VINP_APSReqtest_enum ==
  SignalInput1 : Inport
  SignalInput2 : Inport  Port=2
  VINP_SCPSystemMode_enum : Inport  Port=3
  VVMC_APSActive_flg : Inport  Port=4
  VVMC_ADASActive_flg : Inport  Port=5
  VVMC_CAASActive_flg : Inport  Port=6
  AND : Logic  Inputs=3  AllPortsSameDT=off  OutDataTypeStr=boolean
  Constant1 : Constant  Value=ENUM_SYSMODE_PRODUCT
  Constant3 : Constant  Value=KVMC_APSDevelopeSW_flg
  Equal : RelationalOperator  Operator===  OutDataTypeStr=boolean  RndMeth=Simplest
  OR : Logic  Operator=OR  Inputs=3  AllPortsSameDT=off  OutDataTypeStr=boolean
  Switch : Switch  Criteria=u2 > Threshold
  SignalOutp : Outport
  wires:
  VVMC_ADASActive_flg/1 -> OR/2
  AND/1 -> OR/1
  OR/1 -> Switch/2
  VVMC_APSActive_flg/1 -> AND/3
  Equal/1 -> AND/1
  VINP_SCPSystemMode_enum/1 -> Equal/1
  Switch/1 -> SignalOutp/1
  SignalInput1/1 -> Switch/1
  SignalInput2/1 -> Switch/3
  Constant3/1 -> AND/2
  Constant1/1 -> Equal/2
  VVMC_CAASActive_flg/1 -> OR/3

== system vmc/VMC/APS function/Signal Rounting/Signal Determination VINP_APSStaSystemtest_enum ==
  SignalInput1 : Inport
  SignalInput2 : Inport  Port=2
  VINP_SCPSystemMode_enum : Inport  Port=3
  VVMC_APSActive_flg : Inport  Port=4
  VVMC_ADASActive_flg : Inport  Port=5
  VTQD_GearActualPosn_enum : Inport  Port=6
  VVMC_CAASActive_flg : Inport  Port=7
  AND : Logic  Inputs=3  AllPortsSameDT=off  OutDataTypeStr=boolean
  AND1 : Logic  AllPortsSameDT=off  OutDataTypeStr=boolean
  Constant1 : Constant  Value=ENUM_SYSMODE_PRODUCT
  Constant2 : Constant  Value=ENUM_GEARACTUALPOSN_P
  Constant3 : Constant  Value=KVMC_APSDevelopeSW_flg
  Constant4 : Constant  Value=ENUM_APSSYSTEMSTA_ENABLE
  Constant5 : Constant  Value=KVMC_APSStaSystemOvrd_flg
  Equal : RelationalOperator  Operator===  OutDataTypeStr=boolean  RndMeth=Simplest
  Equal1 : RelationalOperator  Operator===  OutDataTypeStr=boolean  RndMeth=Simplest
  Equal2 : RelationalOperator  Operator===  OutDataTypeStr=boolean  RndMeth=Simplest
  OR : Logic  Operator=OR  Inputs=5  AllPortsSameDT=off  OutDataTypeStr=boolean
  Switch : Switch  Criteria=u2 > Threshold
  SignalOutp : Outport
  wires:
  Constant1/1 -> Equal/2
  Constant3/1 -> AND/2
  SignalInput2/1 -> Switch/3
  SignalInput1/1 -> Switch/1, [VINP_APSStaSystem_enum]
  Switch/1 -> SignalOutp/1
  VINP_SCPSystemMode_enum/1 -> Equal/1
  Equal/1 -> AND/1
  VVMC_APSActive_flg/1 -> AND/3
  OR/1 -> Switch/2
  AND/1 -> OR/1
  VVMC_ADASActive_flg/1 -> OR/2
  VTQD_GearActualPosn_enum/1 -> Equal1/1
  Constant2/1 -> Equal1/2
  Equal1/1 -> AND1/1
  Equal2/1 -> AND1/2
  [VINP_APSStaSystem_enum] -> Equal2/1
  Constant4/1 -> Equal2/2
  AND1/1 -> OR/3
  Constant5/1 -> OR/4
  VVMC_CAASActive_flg/1 -> OR/5

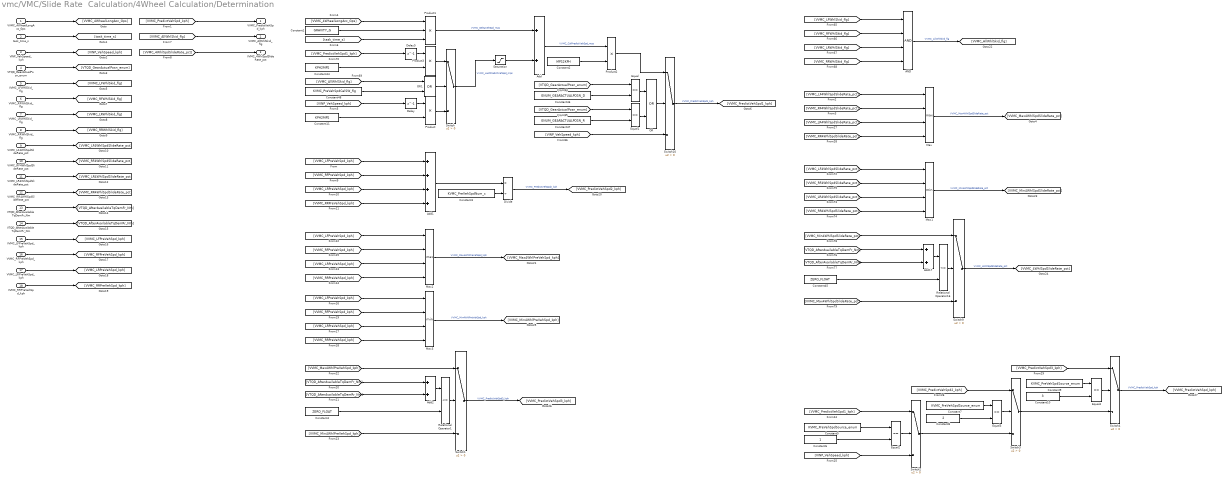
== system vmc/VMC/Slide Rate  Calculation/4Wheel Calculation/Determination ==
  VVMC_4WheelLongAcc_Gps : Inport
  task_time_s : Inport  Port=2
  VINP_VehSpeed_kph : Inport  Port=3
  VTQD_GearActualPosn_enum : Inport  Port=4
  VVMC_LFWhlSkid_flg : Inport  Port=5
  VVMC_RFWhlSkid_flg : Inport  Port=6
  VVMC_LRWhlSkid_flg : Inport  Port=7
  VVMC_RRWhlSkid_flg : Inport  Port=8
  VVMC_LF4WhlSpdSlideRate_pct : Inport  Port=9
  VVMC_RF4WhlSpdSlideRate_pct : Inport  Port=10
  VVMC_LR4WhlSpdSlideRate_pct : Inport  Port=11
  VVMC_RR4WhlSpdSlideRate_pct : Inport  Port=12
  VTQD_AfterAvailableTqDemFr_Nm : Inport  Port=13
  VTQD_AfterAvailableTqDemRr_Nm : Inport  Port=14
  VVMC_LFPreVehSpd_kph : Inport  Port=15
  VVMC_RFPreVehSpd_kph : Inport  Port=16
  VVMC_LRPreVehSpd_kph : Inport  Port=17
  VVMC_RRPreVehSpd_kph : Inport  Port=18
  AND : Logic  Inputs=4  AllPortsSameDT=off  OutDataTypeStr=boolean
  Add : Sum
  Add1 : Sum  Inputs=++++
  Add17 : Sum
  Add2 : Sum
  Constant1 : Constant  Value=GRAVITY_G
  Constant10 : Constant  Value=3
  Constant11 : Constant  Value=KPH2MPS
  Constant2 : Constant  Value=MPS2KPH
  Constant3 : Constant  Value=KVMC_PreVehSpdNum_c
  Constant4 : Constant  Value=ZERO_FLOAT
  Constant44 : Constant  Value=KPH2MPS
  Constant45 : Constant  Value=ZERO_FLOAT
  Constant46 : Constant  Value=ENUM_GEARACTUALPOSN_D
  Constant47 : Constant  Value=ENUM_GEARACTUALPOSN_R
  Constant48 : Constant  Value=KVMC_PreVehSpdCalSW_flg
  Constant5 : Constant  Value=KVMC_PreVehSpdSource_enum
  Constant6 : Constant
  Constant7 : Constant  Value=KVMC_PreVehSpdSource_enum
  Constant8 : Constant  Value=2
  Constant9 : Constant  Value=KVMC_PreVehSpdSource_enum
  Delay : Delay  DelayLength=1
  Delay5 : Delay  DelayLength=1
  Divide : Product  Inputs=*/
  Equal{,1..4} (5 alike) : RelationalOperator  Operator===  OutDataTypeStr=boolean  RndMeth=Simplest
  Max : MinMax  Function=max  Inputs=4
  Max1 : MinMax  Inputs=4
  Max2 : MinMax  Function=max  Inputs=4
  Max3 : MinMax  Inputs=4
  OR : Logic  Operator=OR  AllPortsSameDT=off  OutDataTypeStr=boolean
  OR1 : Logic  Operator=OR  AllPortsSameDT=off  OutDataTypeStr=boolean
  Product : Product
  Product1 : Product  Inputs=3
  Product2 : Product
  Product3 : Product
  Relational Operator1 : RelationalOperator  Operator=<=  OutDataTypeStr=boolean  RndMeth=Simplest
  Relational Operator16 : RelationalOperator  Operator=<=  OutDataTypeStr=boolean  RndMeth=Simplest
  Saturation : Saturate  UpperLimit=KVMC_PredVehSpdLimit_mps  LowerLimit=ZERO_FLOAT
  Switch{,1..4,9..10} (7 alike) : Switch  Criteria=u2 > Threshold
  VVMC_PredictVehSpd_kph : Outport
  VVMC_AllWhlSkid_flg : Outport  Port=2
  VVMC_4WhlSpdSlideRate_pct : Outport  Port=3
  wires:
  [VVMC_RRWhlSkid_flg] -> AND/4
  Add/1 -> Product2/1  "VVMC_CalPredictVehSpd_mps"
  Product2/1 -> Switch10/1
  Relational Operator16/1 -> Switch9/2
  [VVMC_LRWhlSkid_flg] -> AND/3
  Constant45/1 -> Relational Operator16/2
  Switch9/1 -> [VVMC_4WhlSpdSlideRate_pct]  "VVMC_4WhlSpdSlideRate_pct"
  Constant11/1 -> Product/2
  [VVMC_LFWhlSkid_flg] -> AND/1
  [VTQD_GearActualPosn_enum] -> Equal1/1
  Constant2/1 -> Product2/2
  Equal/1 -> OR/1
  AND/1 -> [VVMC_AllWhlSkid_flg]  "VVMC_AllWhlSkid_flg"
  Switch10/1 -> [VVMC_PredictVehSpd1_kph]  "VVMC_PredictVehSpd1_kph"
  Constant1/1 -> Product1/2
  [VINP_VehSpeed_kph] -> Switch10/3
  [VVMC_RF4WhlSpdSlideRate_pct] -> Max/2
  [VINP_VehSpeed_kph] -> Delay/1
  [task_time_s] -> Product1/3
  [VVMC_AllWhlSkid_flg] -> OR1/1
  [VVMC_RR4WhlSpdSlideRate_pct] -> Max/4
  OR/1 -> Switch10/2
  Switch/1 -> Saturation/1  "VVMC_LastPredictVehSpd_mps"
  Product/1 -> Switch/3
  Product3/1 -> Switch/1
  Delay5/1 -> Product3/1
  [VVMC_LR4WhlSpdSlideRate_pct] -> Max/3
  [VVMC_4WheelLongAcc_Gps] -> Product1/1
  [VVMC_LF4WhlSpdSlideRate_pct] -> Max1/1
  [VTQD_AfterAvailableTqDemRr_Nm] -> Add17/2
  [VVMC_LF4WhlSpdSlideRate_pct] -> Max/1
  [VVMC_RFWhlSkid_flg] -> AND/2
  [VVMC_Max4WhlSpdSlideRate_pct] -> Switch9/3
  Max1/1 -> [VVMC_Min4WhlSpdSlideRate_pct]  "VVMC_Min4WhlSpdSlideRate_pct"
  Saturation/1 -> Add/2
  [VTQD_GearActualPosn_enum] -> Equal/1
  [VVMC_RR4WhlSpdSlideRate_pct] -> Max1/4
  [VTQD_AfterAvailableTqDemFr_Nm] -> Add17/1
  OR1/1 -> Switch/2
  Product1/1 -> Add/1  "VVMC_DeltaVehSpd_mps"
  Constant46/1 -> Equal/2
  Delay/1 -> Product/1
  [VVMC_RF4WhlSpdSlideRate_pct] -> Max1/2
  Equal1/1 -> OR/2
  [VVMC_Min4WhlSpdSlideRate_pct] -> Switch9/1
  Constant47/1 -> Equal1/2
  Add17/1 -> Relational Operator16/1
  Max/1 -> [VVMC_Max4WhlSpdSlideRate_pct]  "VVMC_Max4WhlSpdSlideRate_pct"
  Constant44/1 -> Product3/2
  Constant48/1 -> OR1/2
  [VVMC_LR4WhlSpdSlideRate_pct] -> Max1/3
  VINP_VehSpeed_kph/1 -> [VINP_VehSpeed_kph]
  task_time_s/1 -> [task_time_s]
  VVMC_4WheelLongAcc_Gps/1 -> [VVMC_4WheelLongAcc_Gps]
  VTQD_GearActualPosn_enum/1 -> [VTQD_GearActualPosn_enum]
  [VVMC_PredictVehSpd_kph] -> VVMC_PredictVehSpd_kph/1
  [VVMC_AllWhlSkid_flg] -> VVMC_AllWhlSkid_flg/1
  [VVMC_4WhlSpdSlideRate_pct] -> VVMC_4WhlSpdSlideRate_pct/1
  VVMC_LFWhlSkid_flg/1 -> [VVMC_LFWhlSkid_flg]
  VVMC_RFWhlSkid_flg/1 -> [VVMC_RFWhlSkid_flg]
  VVMC_LRWhlSkid_flg/1 -> [VVMC_LRWhlSkid_flg]
  VVMC_RRWhlSkid_flg/1 -> [VVMC_RRWhlSkid_flg]
  VVMC_LF4WhlSpdSlideRate_pct/1 -> [VVMC_LF4WhlSpdSlideRate_pct]
  VVMC_RF4WhlSpdSlideRate_pct/1 -> [VVMC_RF4WhlSpdSlideRate_pct]
  VVMC_LR4WhlSpdSlideRate_pct/1 -> [VVMC_LR4WhlSpdSlideRate_pct]
  VVMC_RR4WhlSpdSlideRate_pct/1 -> [VVMC_RR4WhlSpdSlideRate_pct]
  VTQD_AfterAvailableTqDemFr_Nm/1 -> [VTQD_AfterAvailableTqDemFr_Nm]
  VTQD_AfterAvailableTqDemRr_Nm/1 -> [VTQD_AfterAvailableTqDemRr_Nm]
  VVMC_LFPreVehSpd_kph/1 -> [VVMC_LFPreVehSpd_kph]
  VVMC_RFPreVehSpd_kph/1 -> [VVMC_RFPreVehSpd_kph]
  VVMC_LRPreVehSpd_kph/1 -> [VVMC_LRPreVehSpd_kph]
  VVMC_RRPreVehSpd_kph/1 -> [VVMC_RRPreVehSpd_kph]
  [VVMC_LFPreVehSpd_kph] -> Add1/1
  [VVMC_RFPreVehSpd_kph] -> Add1/2
  [VVMC_LRPreVehSpd_kph] -> Add1/3
  [VVMC_RRPreVehSpd_kph] -> Add1/4
  Add1/1 -> Divide/1
  Constant3/1 -> Divide/2
  Divide/1 -> [VVMC_PredictVehSpd2_kph]  "VVMC_PredictVehSpd2_kph"
  [VVMC_LFPreVehSpd_kph] -> Max2/1
  [VVMC_RFPreVehSpd_kph] -> Max2/2
  [VVMC_LRPreVehSpd_kph] -> Max2/3
  [VVMC_RRPreVehSpd_kph] -> Max2/4
  Max2/1 -> [VVMC_Max4WhlPreVehSpd_kph]  "VVMC_Max4WhlPreVehSpd_kph"
  [VVMC_RRPreVehSpd_kph] -> Max3/4
  [VVMC_LRPreVehSpd_kph] -> Max3/3
  [VVMC_RFPreVehSpd_kph] -> Max3/2
  [VVMC_LFPreVehSpd_kph] -> Max3/1
  Max3/1 -> [VVMC_Min4WhlPreVehSpd_kph]  "VVMC_Min4WhlPreVehSpd_kph"
  Relational Operator1/1 -> Switch1/2
  Constant4/1 -> Relational Operator1/2
  Add2/1 -> Relational Operator1/1
  Switch1/1 -> [VVMC_PredictVehSpd3_kph]  "VVMC_PredictVehSpd3_kph"
  [VVMC_PredictVehSpd1_kph] -> Delay5/1
  Constant5/1 -> Equal2/1
  Constant6/1 -> Equal2/2
  Equal2/1 -> Switch2/2
  [VVMC_PredictVehSpd1_kph] -> Switch2/1
  [VINP_VehSpeed_kph] -> Switch2/3
  Equal3/1 -> Switch3/2
  Constant8/1 -> Equal3/2
  Constant7/1 -> Equal3/1
  Switch2/1 -> Switch3/3
  [VVMC_PredictVehSpd2_kph] -> Switch3/1
  Switch3/1 -> Switch4/3
  Constant9/1 -> Equal4/1
  Constant10/1 -> Equal4/2
  Equal4/1 -> Switch4/2
  [VVMC_PredictVehSpd3_kph] -> Switch4/1
  Switch4/1 -> [VVMC_PredictVehSpd_kph]  "VVMC_PredictVehSpd_kph"
  [VTQD_AfterAvailableTqDemFr_Nm] -> Add2/1
  [VTQD_AfterAvailableTqDemRr_Nm] -> Add2/2
  [VVMC_Max4WhlPreVehSpd_kph] -> Switch1/1
  [VVMC_Min4WhlPreVehSpd_kph] -> Switch1/3

== system vmc/VMC/Slide Rate  Calculation/4Wheel Calculation/LF Wheel ==
  VVMC_4WheelLongAcc_Gps : Inport
  task_time_s : Inport  Port=2
  VINP_LFRawWhlSpeed_kph : Inport  Port=3
  VTQD_GearActualPosn_enum : Inport  Port=4
  AND1 : Logic  Inputs=3  AllPortsSameDT=off  OutDataTypeStr=boolean
  Abs : Abs
  Add : Sum
  Add{1,5,9..10} (4 alike) : Sum  Inputs=+-
  Constant1 : Constant  Value=GRAVITY_G
  Constant11 : Constant  Value=KPH2MPS
  Constant2 : Constant  Value=MPS2KPH
  Constant24 : Constant  Value=KPH2MPS
  Constant25 : Constant  Value=GRAVITY_G
  Constant26 : Constant  Value=KVMC_WhlSpdCalAccTs_c
  Constant3 : Constant  Value=KVMC_4WheelEnSkidDetSpd_kph
  Constant36 : Constant  Value=KVMC_WheelSkidAccDev_Gps
  Constant37 : Constant  Value=KVMC_SkidRecVehSpdDev_kph
  Constant44 : Constant  Value=KPH2MPS
  Constant46 : Constant  Value=ENUM_GEARACTUALPOSN_D
  Constant47 : Constant  Value=ENUM_GEARACTUALPOSN_R
  Constant48 : Constant  Value=KVMC_PreVehSpdCalSW_flg
  Constant5 : Constant  Value=KVMC_RawWhlSpeedDeadZone_kph
  Constant52 : Constant  Value=KVMC_LFWhlSkidReset_flg
  Constant6 : Constant  Value=ONE_FLOAT
  Constant7 : Constant  Value=ONE_PERCENT
  Constant8 : Constant  Value=KVMC_RawWhlSpeedDeadZone_kph
  Constant9 : Constant  Value=ZERO_FLOAT
  Delay{,1,5..7,14} (6 alike) : Delay  DelayLength=1
  Divide : Product  Inputs=**//
  Divide1 : Product  Inputs=*//
  Equal : RelationalOperator  Operator===  OutDataTypeStr=boolean  RndMeth=Simplest
  Equal1 : RelationalOperator  Operator===  OutDataTypeStr=boolean  RndMeth=Simplest
  FirstOrderFilter : hcu_lib/Basic_Blocks/FirstOrderFilter
  OR : Logic  Operator=OR  AllPortsSameDT=off  OutDataTypeStr=boolean
  OR1 : Logic  Operator=OR  AllPortsSameDT=off  OutDataTypeStr=boolean
  OR2 : Logic  Operator=OR  AllPortsSameDT=off  OutDataTypeStr=boolean
  Product : Product
  Product1 : Product  Inputs=3
  Product2 : Product
  Product3 : Product
  Relational Operator : RelationalOperator  Operator=>  OutDataTypeStr=boolean  RndMeth=Simplest
  Relational Operator{1..3,9} (4 alike) : RelationalOperator  Operator=<=  OutDataTypeStr=boolean  RndMeth=Simplest
  SR_Latch : hcu_lib/Basic_Blocks/SR_Latch
  Saturation : Saturate  UpperLimit=KVMC_PredVehSpdLimit_mps  LowerLimit=ZERO_FLOAT
  Switch{,2..3,10} (4 alike) : Switch  Criteria=u2 > Threshold
  VVMC_LFPreVehSpd_kph : Outport
  VVMC_LFWhlSkid_flg : Outport  Port=2
  VVMC_LF4WhlSpdSlideRate_pct : Outport  Port=3
  wires:
  [VINP_LFRawWhlSpeed_kph] -> Delay7/1
  Constant37/1 -> Relational Operator9/2
  Relational Operator9/1 -> AND1/1
  Constant9/1 -> Switch3/1
  Constant36/1 -> Relational Operator/2
  Constant52/1 -> AND1/3
  Constant8/1 -> Relational Operator3/2
  Constant6/1 -> Switch2/1
  Delay14/1 -> AND1/2
  Abs/1 -> Relational Operator9/1
  [VVMC_4WheelLongAcc_Gps] -> Add9/2
  [VVMC_LFWhlSkid_flg] -> Delay14/1
  Relational Operator3/1 -> Switch3/2
  Add10/1 -> Abs/1
  [task_time_s] -> FirstOrderFilter/2
  Constant26/1 -> FirstOrderFilter/3
  Delay6/1 -> Add10/1
  SR_Latch/1 -> [VVMC_LFWhlSkid_flg]  "VVMC_LFWhlSkid_flg"
  Divide1/1 -> Switch3/3  "VVMC_LFCal4WhlSpdSlideRate_pct"
  [VINP_LFRawWhlSpeed_kph] -> Add5/1
  [VVMC_LFPreVehSpd_kph] -> Add1/2
  Switch2/1 -> Divide1/3
  Relational Operator2/1 -> Switch2/2
  Divide/1 -> FirstOrderFilter/1
  [VVMC_LFWhlCalAcc_Gps] -> Add9/1
  [VVMC_LFPreVehSpd_kph] -> Relational Operator2/1
  Constant5/1 -> Relational Operator2/2
  Add9/1 -> Relational Operator/1
  Switch3/1 -> [VVMC_LF4WhlSpdSlideRate_pct]  "VVMC_LF4WhlSpdSlideRate_pct"
  Relational Operator/1 -> SR_Latch/1
  Add1/1 -> Divide1/1
  Delay7/1 -> Add10/2
  Constant7/1 -> Divide1/2
  [VVMC_LFPreVehSpd_kph] -> Switch2/3
  [VINP_LFRawWhlSpeed_kph] -> Add1/1
  Delay1/1 -> Add5/2
  [VINP_LFRawWhlSpeed_kph] -> Relational Operator3/1
  [task_time_s] -> Divide/3
  Constant25/1 -> Divide/4
  Constant24/1 -> Divide/2
  [VINP_LFRawWhlSpeed_kph] -> Delay1/1
  Add5/1 -> Divide/1
  FirstOrderFilter/1 -> [VVMC_LFWhlCalAcc_Gps]  "VVMC_LFWhlCalAcc_Gps"
  Constant48/1 -> OR1/2
  Constant44/1 -> Product3/2
  Switch10/1 -> [VVMC_LFPreVehSpd_kph]  "VVMC_LFPreVehSpd_kph"
  Constant47/1 -> Equal1/2
  Product2/1 -> Switch10/1
  OR1/1 -> Switch/2
  Equal1/1 -> OR/2
  Constant46/1 -> Equal/2
  Product1/1 -> Add/1  "VVMC_LFDeltaVehSpd_mps"
  Saturation/1 -> Add/2
  [VTQD_GearActualPosn_enum] -> Equal1/1
  Delay/1 -> Product/1
  [VINP_LFRawWhlSpeed_kph] -> Switch10/3
  [VTQD_GearActualPosn_enum] -> Equal/1
  OR/1 -> Switch10/2
  [VVMC_4WheelLongAcc_Gps] -> Product1/1
  Product3/1 -> Switch/1
  Delay5/1 -> Product3/1
  Product/1 -> Switch/3
  Switch/1 -> Saturation/1  "VVMC_LFLastPreVehSpd_mps"
  Constant2/1 -> Product2/2
  Equal/1 -> OR/1
  Constant1/1 -> Product1/2
  Constant11/1 -> Product/2
  [task_time_s] -> Product1/3
  Add/1 -> Product2/1  "VVMC_LFCalPreVehSpd_mps"
  [VVMC_LFPreVehSpd_kph] -> Delay5/1
  [VINP_LFRawWhlSpeed_kph] -> Delay/1
  [VVMC_LFPreVehSpd_kph] -> Delay6/1
  VVMC_4WheelLongAcc_Gps/1 -> [VVMC_4WheelLongAcc_Gps]
  task_time_s/1 -> [task_time_s]
  VINP_LFRawWhlSpeed_kph/1 -> [VINP_LFRawWhlSpeed_kph]
  [VVMC_LFWhlSkid_flg] -> OR1/1
  VTQD_GearActualPosn_enum/1 -> [VTQD_GearActualPosn_enum]
  [VVMC_LFPreVehSpd_kph] -> VVMC_LFPreVehSpd_kph/1
  [VVMC_LFWhlSkid_flg] -> VVMC_LFWhlSkid_flg/1
  [VVMC_LF4WhlSpdSlideRate_pct] -> VVMC_LF4WhlSpdSlideRate_pct/1
  OR2/1 -> SR_Latch/2  "VVMC_LFWhlSkidReset_flg"
  AND1/1 -> OR2/2
  Relational Operator1/1 -> OR2/1
  Constant3/1 -> Relational Operator1/2
  [VINP_LFRawWhlSpeed_kph] -> Relational Operator1/1
